simulink model "model_cnn"  (R2020a)
settings: Solver=VariableStepAuto  StartTime=0.0  StopTime=1e6/fs  RelTol=1e-3
PreLoadFcn:
  | setup_imports;
  | %dense2_numerictype = fixdt(1,18,10);
  | %conv1_numerictype = fixdt(1,18,21);
InitFcn:
  | % Intermediate signal dimensions
  | input_dim = [1, 2, 128];
  | layer1_dim = hInterConvLayerDims([1,3,1,64],input_dim,1); % dims : [C,H,W]
  | layer2_dim = hInterConvLayerDims([2,3,64,16],layer1_dim,1);% dims : [C,H,W]
  | layer3_dim = [1,128];
  | 
  | % Conv Layer 1 dimensions
  | conv1_dims = struct(...
  |     'input_dim',    input_dim,...       input_dim = C,H,W
  |     'filter_dim',   [1, 3, 1, 64],...  filter_dim = K,J,C,N
  |     'stride',       1,...
  |     'row_output',   3,...
  |     'output_dim',   layer1_dim);
  | 
  | % Conv Layer 2 dimensions
  | conv2_dims = struct(...
  |     'input_dim',    layer1_dim,...      input = C,H.W
  |     'filter_dim',   [2, 3, 64, 16],...  filter_dim = K,J,C,N
  |     'stride',       1,...
  |     'row_output',   2*3*64,...
  |     'output_dim',   layer2_dim);
  | 
  | % Dense Layer 1 dimensions
  | dense1_dims = struct(...
  |     'input_dim',    layer2_dim,...      input = C,H,W
  |     'weight_dim',   [1984, 128],...     weight_dim = H,W
  |     'output_dim',   layer3_dim);
  | 
  | % Load saved weights and input
  | setup_imports;
  | 
  | fs = 128e6;
  | fs_axi = 100e6;
  | R = 32;
values from neighbouring files (symbols this model uses):
  datatypeInput = X_test.numerictype    [setup_imports.m]
  gemm_wconv1 = fi(hInterleaveFilters(Wconv1),1,16)    [setup_imports.m]
  gemm_wconv2 = fi(hInterleaveFilters(Wconv2),1,16)    [setup_imports.m]
  wdense1 = fi(Wdense1,1,16)    [setup_imports.m]
  wdense2 = fi(Wdense2,1,16)    [setup_imports.m]
undefined symbols (not defined in the file or in its folder): ltehdlRAMinitPO2
libraries: hdlsllib x1022, dspsigops x3, dspsrcs4 x2
(part 23 of 23)

== matlab function model_cnn/HDL CNN Model/Dense Layer 2/Output Buffer3 ==
  data: vectorIn input; samplesOut output; validIn input; validOut output; done output boolean
function [samplesOut, validOut, done]  = output_buffer(vectorIn, validIn)

    vector_size = 8;
    persistent reg buffer
    
    if isempty(reg)
        reg = struct(...
            'validOut',     false,...
            'flag',         false,...
            'count_out',    fi(0,0,ceil(log2(vector_size))+1,0,hdlfimath));   % for a vector of 16
    end
    
    if isempty(buffer)
%         buffer = fi(zeros(vector_size,1),1,16,15);
        buffer = cast(zeros(vector_size,1),'like',vectorIn);
    end

    if validIn
        reg.flag = true;
        buffer(:) = vectorIn;
        reg.count_out(:) = 0;
    end
    
    done = logical(false);
    
    if reg.flag
        samplesOut = buffer(reg.count_out+1);
        reg.count_out(:) = reg.count_out + 1;
        validOut = true;
        if reg.count_out == vector_size
            reg.flag = false;
            done = true;
        end
    else
        reg.count_out(:) = 0;
        reg.flag = false;
        samplesOut = cast(0,'like',vectorIn);
%         samplesOut = fi(0,vectorIn.numerictype);
        validOut = false;
    end
    
end

== matlab function model_cnn/HDL CNN Model/Collect Input into Bursts/Ping Pong Buffer Controller ==
  data: wr_en0 output; wr_en1 output; bufferSelect output; ram0_addr output; ram1_addr output; validIn input; validOut output
function [wr_en0, wr_en1, bufferSelect, ram0_addr, ram1_addr, validOut] = PPBufferCounter(validIn)
    persistent reg state;
    INITIAL_STATE = 0;
    FIRST_WRITE = 1;
    READ_PING = 2;
    READ_PONG = 3;
    
    ADDR_LENGTH = 256;
    
    if isempty(reg)
        reg = struct('wr_count',                fi(0,0,ceil(log2(ADDR_LENGTH))+1,0,hdlfimath),...
                     'rd_count',                fi(0,0,ceil(log2(ADDR_LENGTH))+1,0,hdlfimath),...
                     'bufferSwitch',            false,...
                     'flag_first_write',        false,...
                     'flag_read_ping',          true,...
                     'flag_write_ping',         false,...
                     'flag_read_pong',          true,...
                     'flag_write_pong',         false,...
                     'wr_en0',                  false,...
                     'wr_en1',                  false);
    end
    
    if isempty(state)
        state = fi(INITIAL_STATE,0,4,0);
    end
    
    bufferSelect = false;
    wr_en0 = false;
    wr_en1 = false;
    ram0_addr = fi(0,0,ceil(log2(ADDR_LENGTH))+1,0,hdlfimath);
    ram1_addr = fi(0,0,ceil(log2(ADDR_LENGTH))+1,0,hdlfimath);
    validOut = false;
    
    switch state
        case INITIAL_STATE
            if validIn
                state(:) = FIRST_WRITE;
                reg.wr_en0 = true;
                reg.wr_count(:) = reg.wr_count + 1;
            else
                reg.wr_en0 = false;                
            end
            wr_en0 = reg.wr_en0;
        case FIRST_WRITE
            if validIn
                if reg.wr_count == ADDR_LENGTH - 1
                    reg.flag_first_write = true;
                    ram0_addr = reg.wr_count;
                    reg.wr_count(:) = 0;
                else
                    ram0_addr = reg.wr_count;
                    reg.wr_count(:) = reg.wr_count + 1;
                end
                reg.wr_en0 = true;
            else
                reg.wr_en0 = false;
            end
            wr_en0 = reg.wr_en0;
            
            if reg.flag_first_write
                state(:) = READ_PING;
                reg.rd_count(:) = 0;
                reg.wr_count(:) = 0;
            end
            
        case READ_PING
            if reg.flag_read_ping
                if reg.rd_count == ADDR_LENGTH - 1
                    reg.flag_read_ping = false;
                    ram0_addr = reg.rd_count;
                    reg.rd_count(:) = 0;
                else
                    ram0_addr = reg.rd_count;
                    reg.rd_count(:) = reg.rd_count + 1;
                end
                validOut = true;
            end
            bufferSelect = false;
            reg.wr_en0 = false;
            wr_en0 = reg.wr_en0;
            if validIn
                if reg.wr_count == ADDR_LENGTH - 1
                    reg.flag_write_ping = true;
                    ram1_addr = reg.wr_count;
                    reg.wr_count(:) = 0;
                else
                    ram1_addr = reg.wr_count;
                    reg.wr_count(:) = reg.wr_count + 1;
                end
                reg.wr_en1 = true;
            else
                reg.wr_en1 = false;
            end
            wr_en1 = reg.wr_en1;
            
            if reg.flag_write_ping && ~reg.flag_read_ping
                state(:) = READ_PONG;
                reg.flag_write_ping = false;
                reg.flag_read_ping = true;
                reg.rd_count(:) = 0;
                reg.wr_count(:) = 0;
            end
            
        case READ_PONG
            if reg.flag_read_pong
                if reg.rd_count == ADDR_LENGTH - 1
                    reg.flag_read_pong = false;
                    ram1_addr = reg.rd_count;
                    reg.rd_count(:) = 0;
                else
                    ram1_addr = reg.rd_count;
                    reg.rd_count(:) = reg.rd_count + 1;
                end
                validOut = true;
            end
            bufferSelect = true;
            reg.wr_en1 = false;
            wr_en1 = reg.wr_en1;
            if validIn
                if reg.wr_count == ADDR_LENGTH - 1
                    reg.flag_write_pong = true;
                    ram0_addr = reg.wr_count;
                    reg.wr_count(:) = 0;
                else
                    ram0_addr = reg.wr_count;
                    reg.wr_count(:) = reg.wr_count + 1;
                end
                reg.wr_en0 = true;
            else
                reg.wr_en0 = false;
            end
            
            wr_en0 = reg.wr_en0;
            
            if reg.flag_write_pong && ~reg.flag_read_pong
                state(:) = READ_PING;
                reg.flag_write_pong = false;
                reg.flag_read_pong = true;
                reg.rd_count(:) = 0;
                reg.wr_count(:) = 0;
            end
    end
end
